simulink model "Week2_Problem3"  (R2020b)
settings: Solver=VariableStepAuto  StartTime=0.0  StopTime=120  RelTol=1e-3
PostLoadFcn:
  | Kp= 350
  | Kd=300
  | Ki=50
model workspace (MAT data in the model file):
  Kd = 300
  Ki = 50
  Kp = 350
  b = 50
  m = 1000
  u = 500
settings Model: Creator=sai  LastModifiedBy=sai

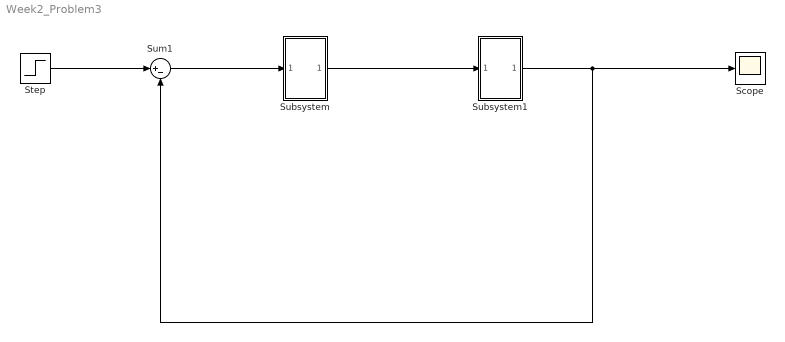
== system Week2_Problem3 ==
  Scope : Scope
  Step : Step  Time=0  After=u  SampleTime=0
  Subsystem : ModelReference  ModelNameDialog=Subsystem  ModelReferenceVersion=1.1
  Subsystem1 : ModelReference  ModelNameDialog=Subsystem1  ModelReferenceVersion=1.1
  Sum1 : Sum  Inputs=|+-
  wires:
  Step/1 -> Sum1/1
  Sum1/1 -> Subsystem/1
  Subsystem/1 -> Subsystem1/1
  Subsystem1/1 -> Sum1/2, Scope/1
